simulink model "signalLogging"  (R2016b)
settings: Solver=VariableStepAuto  StartTime=0.0  StopTime=10  RelTol=1e-3
settings Model: Creator=vibek  LastModifiedBy=vibek

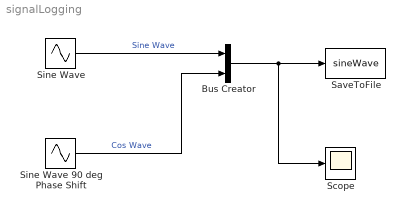
== system signalLogging ==
  Bus Creator : BusCreator  Inputs=2
  SaveToFile : ToFile  Filename=sineWave  MatrixName=result  SaveFormat=Timeseries
  Scope : Scope
  Sine Wave : Sin  Amplitude=5  SampleTime=0
  Sine Wave 90 deg Phase Shift : Sin  Amplitude=5  Phase=1.5708  SampleTime=0
  wires:
  Sine Wave 90 deg Phase Shift/1 -> Bus Creator/2  "Cos Wave"
  Sine Wave/1 -> Bus Creator/1  "Sine Wave"
  Bus Creator/1 -> Scope/1, SaveToFile/1
